simulink model "one_time_switch_test"  (R2019a)
settings: Solver=VariableStepAuto  StartTime=0.0  StopTime=10.0  RelTol=1e-3
settings Model: Creator=asmialek  LastModifiedBy=asmialek

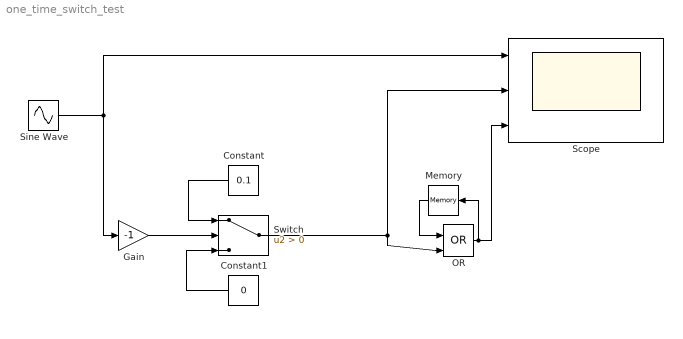
== system one_time_switch_test ==
  Constant : Constant  Value=0.1
  Constant1 : Constant  Value=0
  Gain : Gain  Gain=-1
  Memory : Memory
  OR : Logic  Operator=OR  IconShape=distinctive  AllPortsSameDT=off  OutDataTypeStr=boolean
  Scope : Scope  NumInputPorts=3
  Sine Wave : Sin  SampleTime=0
  Switch : Switch  Criteria=u2 > Threshold
  wires:
  Sine Wave/1 -> Scope/1, Gain/1
  Constant1/1 -> Switch/3
  Constant/1 -> Switch/1
  Switch/1 -> OR/2, Scope/2
  Gain/1 -> Switch/2
  OR/1 -> Memory/1, Scope/3
  Memory/1 -> OR/1
